simulink model "GolfSwing3D_KineticallyDrivenVariantSubsystems"  (R2024b)
settings: Solver=VariableStepAuto  StartTime=0.0  StopTime=StopTime  MaxStep=0.001  RelTol=1e-3
model workspace: external: MAT-File 3DModelInputs.mat (data not in the file)
undefined symbols (not defined in the file or in its folder): GripStrength, KillswitchFinalValue, KillswitchInitialValue, KillswitchStepTime, LeftLowerArmLength, PlaneTilt, RightLowerArmLength, UpperTorsoLength, X, Y, Z
libraries: nesl_utility x355, sm_lib x136, matrix_library x11, simulink x1
(part 1 of 13)
settings Model: Creator=dolso  LastModifiedBy=diete
settings SolverCC: MaxConsecutiveMinStep=20
settings DataIOCC: SaveOutput=off  SaveState=on
settings OptimizationCC: ReuseModelBlockBuffer=off
settings RTWCC: GPUComputeCapability=3.5
settings SimscapeCC: SimscapeLogType=all  SimscapeLogSimulationStatistics=on  SimscapeLogLimitData=off
settings ExplorerConfigSet: InternalSimMechanicsExplorerSettings="<ExplorerConfiguration><canonicalview>default</canonicalview><AnimationSetting><BasePlaybackSpeed>1.0</BasePlaybackSpeed><PlaybackSpeedFactor>1.0</PlaybackSpeedFactor></AnimationSetting><TilePanel><TileInfo><Tiles Columns=\"1\" Count=\"1\" Rows=\"1\"><Column Weight=\"1\"/><Row Weight=\"1\"/><Tile Height=\"1\" Width=\"1\" X=\"0\" Y=\"0\"/></Tiles></TileInfo><SceneInfo><SceneViewer><BGColor><R>0.800000011920928955</R><G>1</G><B>0.800000011920928955</B></BGColor><Camera><DoPerspective>off</DoPerspective><Position><X>0.223338250481492168</X><Y>-2.01724941781281597</Y><Z>0.561965888227227262</Z></Position><Center><X>0.223338250481492168</X><Y>-0.356681108474731556</Y><Z>0.561965888227227262</Z></Center><Up><X>0</X><Y>-0</Y><Z>1</Z></Up><ViewLimDist>1</ViewLimDist><YLim>1.48392906746005671</YLim><XLim>2.01139200613069313</XLim></Camera></SceneViewer></SceneInfo></TilePanel><MechEditorPanel><Cameras/><GfxPanelCameraMap/><VideoCreator><PlaybackSpeedRatio>1.0</PlaybackSpeedRatio><FrameRate>30</FrameRate><VideoFormat>Motion JPEG AVI</VideoFormat><FrameSize>auto</FrameSize></VideoCreator></MechEditorPanel></ExplorerConfiguration>"

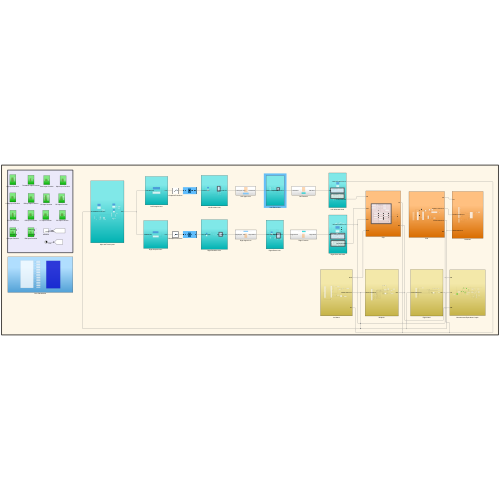
[thumbnail: Simulink's stored preview of the top-level diagram]
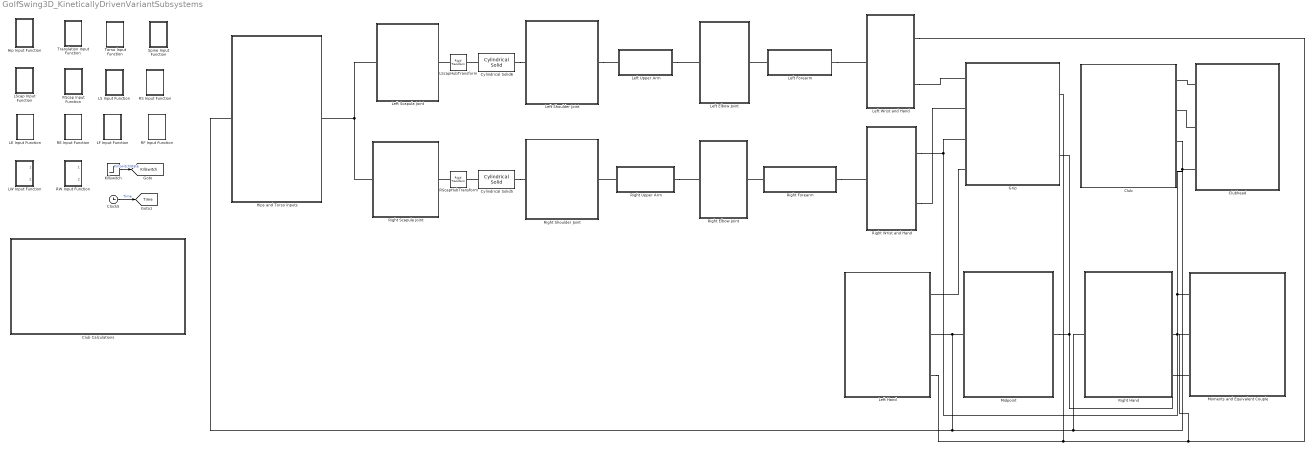
== system GolfSwing3D_KineticallyDrivenVariantSubsystems ==
  Clock5 : Clock
  Club : Subsystem
  Club Calculations : Subsystem
  Clubhead : Subsystem
  Cylindrical Solid5 : sm_lib/Body Elements/Cylindrical Solid  CylinderRadius=3  CylinderRadiusUnits=in  CylinderLength=10  CylinderLengthUnits=in  ExportEntireGeometry=off  InertiaType=CalculateFromGeometry  BasedOnType=Mass  Density=2000  DensityUnits=kg/m^3  Mass=10  MassUnits=kg  CenterOfMass=[0 0 0]  CenterOfMassUnits=m  MomentsOfInertia=[1 1 1]  MomentsOfInertiaUnits=kg*m^2  ProductsOfInertia=[0 0 0]  ProductsOfInertiaUnits=kg*m^2  GraphicType=FromGeometry  MarkerShape=Sphere  MarkerSize=10  GraphicVisPropType=SimpleVisualProperties  GraphicDiffuseColor=[0.2 0.2 1.0]  GraphicOpacity=1.0  GraphicSpecularColor=[0.5 0.5 0.5 1.0]  GraphicAmbientColor=[0.15 0.15 0.15 1.0]  GraphicEmissiveColor=[0.0 0.0 0.0 1.0]  GraphicShininess=75  DoExposeReferenceFrame=off  SerializedFrames=<Frames><Frame><Id>Frame1</Id><Value><Name>Hub</Name><Origin><Source>GeometricFeature</Source><FeatureName>top curve</FeatureName></Origin><PrimaryAxis><DefinedDirection>+X</DefinedDirection><Source>ReferenceFrame</Source><SourceDirection>-Z</SourceDirection><FeatureName></FeatureName></PrimaryAxis><SecondaryAxis><DefinedDirection>+Z</DefinedDirection><Source>ReferenceFrame</Source><SourceDirection>+Y</SourceDirection><FeatureName></FeatureName></SecondaryAxis></Value></Frame><Frame><Id>Frame2</Id><Value><Name>Right Shoulder</Name><Origin><Source>GeometricFeature</Source><FeatureName>bottom curve</FeatureName></Origin><PrimaryAxis><DefinedDirection>-X</DefinedDirection><Source>ReferenceFrame</Source><SourceDirection>+Z</SourceDirection><FeatureName></FeatureName></PrimaryAxis><SecondaryAxis><DefinedDirection>+Y</DefinedDirection><Source>ReferenceFrame</Source><SourceDirection>+X</SourceDirection><FeatureName></FeatureName></SecondaryAxis></Value></Frame></Frames>
  Cylindrical Solid6 : sm_lib/Body Elements/Cylindrical Solid  CylinderRadius=3  CylinderRadiusUnits=in  CylinderLength=10  CylinderLengthUnits=in  ExportEntireGeometry=off  InertiaType=CalculateFromGeometry  BasedOnType=Mass  Density=2000  DensityUnits=kg/m^3  Mass=10  MassUnits=kg  CenterOfMass=[0 0 0]  CenterOfMassUnits=m  MomentsOfInertia=[1 1 1]  MomentsOfInertiaUnits=kg*m^2  ProductsOfInertia=[0 0 0]  ProductsOfInertiaUnits=kg*m^2  GraphicType=FromGeometry  MarkerShape=Sphere  MarkerSize=10  GraphicVisPropType=SimpleVisualProperties  GraphicDiffuseColor=[0.2 0.2 1.0]  GraphicOpacity=1.0  GraphicSpecularColor=[0.5 0.5 0.5 1.0]  GraphicAmbientColor=[0.15 0.15 0.15 1.0]  GraphicEmissiveColor=[0.0 0.0 0.0 1.0]  GraphicShininess=75  DoExposeReferenceFrame=off  SerializedFrames=<Frames><Frame><Id>Frame1</Id><Value><Name>Hub</Name><Origin><Source>GeometricFeature</Source><FeatureName>top curve</FeatureName></Origin><PrimaryAxis><DefinedDirection>+X</DefinedDirection><Source>ReferenceFrame</Source><SourceDirection>-Z</SourceDirection><FeatureName></FeatureName></PrimaryAxis><SecondaryAxis><DefinedDirection>+Z</DefinedDirection><Source>ReferenceFrame</Source><SourceDirection>+Y</SourceDirection><FeatureName></FeatureName></SecondaryAxis></Value></Frame><Frame><Id>Frame2</Id><Value><Name>Left Shoulder</Name><Origin><Source>GeometricFeature</Source><FeatureName>bottom curve</FeatureName></Origin><PrimaryAxis><DefinedDirection>-X</DefinedDirection><Source>ReferenceFrame</Source><SourceDirection>+Z</SourceDirection><FeatureName></FeatureName></PrimaryAxis><SecondaryAxis><DefinedDirection>+Y</DefinedDirection><Source>ReferenceFrame</Source><SourceDirection>+X</SourceDirection><FeatureName></FeatureName></SecondaryAxis></Value></Frame></Frames>
  Grip : Subsystem
  Hip Input Function : Subsystem
  Hips and Torso Inputs : Subsystem
  Killswitch : Step  Time=KillswitchStepTime  Before=KillswitchInitialValue  After=KillswitchFinalValue  SampleTime=0
  LE Input Function : Subsystem
  LF Input Function : Subsystem
  LS Input Function : Subsystem
  LScap Input Function : Subsystem
  LScapHubTransform : sm_lib/Frames and Transforms/Rigid Transform  RotationMethod=RotationSequence  FollAlignAxisA=+X  BaseAlignAxisA=+Y  FollAlignAxisB=+Y  BaseAlignAxisB=+Z  RotationStandardAxis=+Z  RotationAngle=0  RotationAngleUnits=deg  RotationArbitraryAxis=[0 0 1]  RotationSequenceAxes=FollowerAxes  RotationSequence=ZXY  RotationSequenceAngles=[0 0 90]  RotationSequenceAnglesUnits=deg  RotationMatrix=[1 0 0;0 1 0;0 0 1]  Quaternion=[1 0 0 0]  TranslationMethod=None  TranslationCartesianOffset=[0 0 0]  TranslationCartesianOffsetUnits=m  TranslationStandardAxis=+Z  TranslationStandardOffset=0  TranslationStandardOffsetUnits=m  TranslationROffset=0  TranslationROffsetUnits=m  TranslationThetaOffset=0  TranslationThetaOffsetUnits=deg  TranslationZOffset=0  TranslationZOffsetUnits=m
  LW Input Function : Subsystem
  Left Elbow Joint : Subsystem
  Left Forearm : Subsystem
  Left Hand : Subsystem
  Left Scapula Joint : Subsystem
  Left Shoulder Joint : Subsystem
  Left Upper Arm : Subsystem
  Left Wrist and Hand : Subsystem
  Midpoint : Subsystem
  Moments and Equivalent Couple : Subsystem
  RE Input Function : Subsystem
  RF Input Function : Subsystem
  RS Input Function : Subsystem
  RScap Input Function : Subsystem
  RScapHubTransform : sm_lib/Frames and Transforms/Rigid Transform  RotationMethod=RotationSequence  FollAlignAxisA=+X  BaseAlignAxisA=+Y  FollAlignAxisB=+Y  BaseAlignAxisB=+Z  RotationStandardAxis=+Z  RotationAngle=0  RotationAngleUnits=deg  RotationArbitraryAxis=[0 0 1]  RotationSequenceAxes=FollowerAxes  RotationSequence=YXZ  RotationSequenceAngles=[-90 180 0]  RotationSequenceAnglesUnits=deg  RotationMatrix=[1 0 0;0 1 0;0 0 1]  Quaternion=[1 0 0 0]  TranslationMethod=None  TranslationCartesianOffset=[0 0 0]  TranslationCartesianOffsetUnits=m  TranslationStandardAxis=+Z  TranslationStandardOffset=0  TranslationStandardOffsetUnits=m  TranslationROffset=0  TranslationROffsetUnits=m  TranslationThetaOffset=0  TranslationThetaOffsetUnits=deg  TranslationZOffset=0  TranslationZOffsetUnits=m
  RW Input Function : Subsystem
  Right Elbow Joint : Subsystem
  Right Forearm : Subsystem
  Right Hand : Subsystem
  Right Scapula Joint : Subsystem
  Right Shoulder Joint : Subsystem
  Right Upper Arm : Subsystem
  Right Wrist and Hand : Subsystem
  Spine Input Function : Subsystem
  Torso Input Function : Subsystem
  Translation Input Function : Subsystem
  tag scope: Killswitch=global, Time=global
  wires:
  Clock5/1 -> [Time]  "Time"
  Killswitch/1 -> [Killswitch]  "KillswitchState"
  connections:
  Cylindrical Solid6/RConn1 -- Left Shoulder Joint/LConn1
  Left Scapula Joint/LConn1 -- Right Scapula Joint/LConn1 -- Hips and Torso Inputs/LConn1
  LScapHubTransform/LConn1 -- Left Scapula Joint/RConn1
  Cylindrical Solid5/LConn1 -- RScapHubTransform/RConn1
  RScapHubTransform/LConn1 -- Right Scapula Joint/RConn1
  Cylindrical Solid6/LConn1 -- LScapHubTransform/RConn1
  Cylindrical Solid5/RConn1 -- Right Shoulder Joint/LConn1
  Hips and Torso Inputs/RConn1 -- Club/RConn3 -- Clubhead/LConn3 -- Right Hand/LConn1 -- Left Hand/RConn2 -- Midpoint/LConn1
  Left Wrist and Hand/RConn1 -- Left Hand/RConn3 -- Grip/RConn1 -- Moments and Equivalent Couple/LConn2
  Right Wrist and Hand/RConn1 -- Club/RConn4 -- Moments and Equivalent Couple/LConn1 -- Right Hand/RConn1 -- Grip/LConn3
  Left Wrist and Hand/RConn2 -- Grip/LConn1
  Right Wrist and Hand/RConn2 -- Grip/LConn2
  Grip/LConn4 -- Left Hand/RConn1
  Clubhead/LConn1 -- Club/RConn1
  Clubhead/LConn2 -- Club/RConn2
  Midpoint/RConn1 -- Moments and Equivalent Couple/LConn3 -- Grip/RConn2
  Left Shoulder Joint/RConn1 -- Left Upper Arm/LConn1
  Left Upper Arm/RConn1 -- Left Elbow Joint/LConn1
  Left Forearm/LConn1 -- Left Elbow Joint/RConn1
  Left Forearm/RConn1 -- Left Wrist and Hand/LConn1
  Right Upper Arm/LConn1 -- Right Shoulder Joint/RConn1
  Right Upper Arm/RConn1 -- Right Elbow Joint/LConn1
  Right Forearm/LConn1 -- Right Elbow Joint/RConn1
  Right Forearm/RConn1 -- Right Wrist and Hand/LConn1

== system GolfSwing3D_KineticallyDrivenVariantSubsystems/Club ==
  Club COM : nesl_utility/PS-Simulink Converter  PhysicalDomain=network_engine_domain  SubClassName=ps_output  LeftPortType=input  RightPortType=output  PseudoPeriodic=off  Frequencies=[]  VectorFormat=1-D array  Unit=inherit  AffineConversion=off
  Club Mass : nesl_utility/PS-Simulink Converter  PhysicalDomain=network_engine_domain  SubClassName=ps_output  LeftPortType=input  RightPortType=output  PseudoPeriodic=off  Frequencies=[]  VectorFormat=1-D array  Unit=inherit  AffineConversion=off
  Clubface Vector : sm_lib/Body Elements/Cylindrical Solid  CylinderRadius=0.25  CylinderRadiusUnits=in  CylinderLength=CFVectorLength  CylinderLengthUnits=in  ExportEntireGeometry=off  InertiaType=CalculateFromGeometry  BasedOnType=Mass  Density=500  DensityUnits=kg/m^3  Mass=0  MassUnits=g  CenterOfMass=[0 0 0]  CenterOfMassUnits=m  MomentsOfInertia=[1 1 1]  MomentsOfInertiaUnits=kg*m^2  ProductsOfInertia=[0 0 0]  ProductsOfInertiaUnits=kg*m^2  GraphicType=FromGeometry  MarkerShape=Sphere  MarkerSize=10  GraphicVisPropType=SimpleVisualProperties  GraphicDiffuseColor=[0.4941 0.1843 0.5569]  GraphicOpacity=1.0  GraphicSpecularColor=[0.5 0.5 0.5 1.0]  GraphicAmbientColor=[0.15 0.15 0.15 1.0]  GraphicEmissiveColor=[0.0 0.0 0.0 1.0]  GraphicShininess=75  DoExposeReferenceFrame=off  SerializedFrames=<Frames><Frame><Id>Frame1</Id><Value><Name>Club Center</Name><Origin><Source>GeometricFeature</Source><FeatureName>top curve</FeatureName></Origin><PrimaryAxis><DefinedDirection>-Y</DefinedDirection><Source>ReferenceFrame</Source><SourceDirection>+Z</SourceDirection><FeatureName></FeatureName></PrimaryAxis><SecondaryAxis><DefinedDirection>+X</DefinedDirection><Source>ReferenceFrame</Source><SourceDirection>+Y</SourceDirection><FeatureName></FeatureName></SecondaryAxis></Value></Frame><Frame><Id>Frame2</Id><Value><Name>Center of Bottom</Name><Origin><Source>GeometricFeature</Source><FeatureName>bottom surface</FeatureName></Origin><PrimaryAxis><DefinedDirection>+Z</DefinedDirection><Source>ReferenceFrame</Source><SourceDirection>+Z</SourceDirection><FeatureName></FeatureName></PrimaryAxis><SecondaryAxis><DefinedDirection>+X</DefinedDirection><Source>ReferenceFrame</Source><SourceDirection>+X</SourceDirection><FeatureName></FeatureName></SecondaryAxis></Value></Frame></Frames>
  Clubhead : sm_lib/Body Elements/Spherical Solid  SphereRadius=ClubheadRadius  SphereRadiusUnits=in  ExportEntireGeometry=off  InertiaType=CalculateFromGeometry  BasedOnType=Mass  Density=500  DensityUnits=kg/m^3  Mass=0.25  MassUnits=kg  CenterOfMass=[0 0 0]  CenterOfMassUnits=m  MomentsOfInertia=[1 1 1]  MomentsOfInertiaUnits=kg*m^2  ProductsOfInertia=[0 0 0]  ProductsOfInertiaUnits=kg*m^2  GraphicType=FromGeometry  MarkerShape=Sphere  MarkerSize=10  GraphicVisPropType=SimpleVisualProperties  GraphicDiffuseColor=[0.0 0.0 0.0]  GraphicOpacity=1.0  GraphicSpecularColor=[0.5 0.5 0.5 1.0]  GraphicAmbientColor=[0.15 0.15 0.15 1.0]  GraphicEmissiveColor=[0.0 0.0 0.0 1.0]  GraphicShininess=75  DoExposeReferenceFrame=on  SerializedFrames=<Frames/>
  Flexible Beam Model : Subsystem
  ForceonClubhead : nesl_utility/PS-Simulink Converter  Commented=on  PhysicalDomain=network_engine_domain  SubClassName=ps_output  LeftPortType=input  RightPortType=output  PseudoPeriodic=off  Frequencies=[]  VectorFormat=1-D array  Unit=inherit  AffineConversion=off
  GripStrength : sm_lib/Frames and Transforms/Rigid Transform  RotationMethod=RotationSequence  FollAlignAxisA=+X  BaseAlignAxisA=+Y  FollAlignAxisB=+Y  BaseAlignAxisB=+Z  RotationStandardAxis=+Z  RotationAngle=0  RotationAngleUnits=deg  RotationArbitraryAxis=[0 0 1]  RotationSequenceAxes=FollowerAxes  RotationSequence=XYZ  RotationSequenceAngles=[-GripStrength 0 0]  RotationSequenceAnglesUnits=deg  RotationMatrix=[1 0 0;0 1 0;0 0 1]  Quaternion=[1 0 0 0]  TranslationMethod=None  TranslationCartesianOffset=[0 0 0]  TranslationCartesianOffsetUnits=m  TranslationStandardAxis=+Z  TranslationStandardOffset=0  TranslationStandardOffsetUnits=m  TranslationROffset=0  TranslationROffsetUnits=m  TranslationThetaOffset=0  TranslationThetaOffsetUnits=deg  TranslationZOffset=0  TranslationZOffsetUnits=m
  Inertia Sensor : sm_lib/Body Elements/Inertia Sensor  SensorExtent=BodyGroup  SpanWeldJoints=on  ExcludeGroundedBodies=off  MeasurementFrame=World  SenseMass=on  SenseCenterOfMass=on  SenseInertiaMatrix=on  SenseCenteredInertiaMatrix=off  SensePrincipalInertiaMatrix=off  SenseRotationMatrix=off  GraphicType=None  PrincipalInertiaFrameSize=20  GraphicVisPropType=SimpleVisualProperties  GraphicDiffuseColor=[0.5 0.5 0.5]  GraphicOpacity=1.0  GraphicSpecularColor=[0.5 0.5 0.5 1.0]  GraphicAmbientColor=[0.15 0.15 0.15 1.0]  GraphicEmissiveColor=[0.0 0.0 0.0 1.0]  GraphicShininess=75
  Rigid Shaft : Subsystem  Commented=on
  Weld Joint : sm_lib/Joints/Weld Joint  JointMode=Normal  CompositeWrenchDir=BaseOnFollower  CompositeWrenchFrame=BaseFrame  SenseConstraintForce=off  SenseConstraintTorque=off  SenseTotalForce=on  SenseTotalTorque=off
  Zero Mass Reference Shaft : Subsystem
  CH : PMIOPort  Side=Right
  Clubface Reference : PMIOPort  Port=2  Side=Right
  Global Reference : PMIOPort  Port=3  Side=Right
  RH : PMIOPort  Port=4  Side=Right
  tag scope: ClubCOM=global
  wires:
  Club COM/1 -> [ClubCOM]  "ClubCOM"
  ForceonClubhead/1 -> ?  "ForceonClubhead"
  connections:
  ForceonClubhead/LConn1 -- Weld Joint/RConn2
  Inertia Sensor/LConn1 -- CH/RConn1 -- Rigid Shaft/RConn2 -- Flexible Beam Model/RConn1 -- Weld Joint/LConn1
  Inertia Sensor/RConn1 -- Club Mass/LConn1
  Zero Mass Reference Shaft/RConn2 -- Global Reference/RConn1
  Club COM/LConn1 -- Inertia Sensor/RConn2
  GripStrength/LConn1 -- Weld Joint/RConn1
  Clubhead/RConn1 -- Clubface Vector/LConn1 -- GripStrength/RConn1
  Clubface Reference/RConn1 -- Clubface Vector/RConn1
  Zero Mass Reference Shaft/RConn1 -- Flexible Beam Model/LConn1 -- Rigid Shaft/RConn1 -- RH/RConn1

== system GolfSwing3D_KineticallyDrivenVariantSubsystems/Club Calculations ==
  Subsystem : Subsystem
  Work and Impulse Integrators : Subsystem
  tag scope: ForceAlongHandPath=global, ForceonClubMagnitude=global, HandForceYankLocal=global, LHForceAlongHandPath=global, LHonClubAngularPower=global, LHonClubLinearPower=global, LinearPoweronClub=global, RHForceAlongHandPath=global, RHonClubAngularPower=global, RHonClubLinearPower=global, SumofMomentsLHonClub=global, SumofMomentsRHonClub=global, TorqueonClubMagnitude=global, TotalHandForceGlobal=global, TotalHandForceLocal=global, TotalWristTorqueGlobal=global, TotalWristTorqueLocal=global
  wires:
  Subsystem/2(TotalHandTorqueLocal) -> [TotalWristTorqueLocal]  "TotalHandTorqueLocal"
  Subsystem/4(TotalHandTorqueGlobal) -> [TotalWristTorqueGlobal]  "TotalHandTorqueGlobal"
  Subsystem/1(TorqueonClubMagnitude) -> [TorqueonClubMagnitude]  "TorqueonClubMagnitude"
  Subsystem/3(TotalHandForceLocal) -> [TotalHandForceLocal]  "TotalHandForceLocal"
  Subsystem/5(TotalHandForceGlobal) -> [TotalHandForceGlobal]  "TotalHandForceGlobal"
  Subsystem/6(ForceonClubMagnitude) -> [ForceonClubMagnitude]  "ForceonClubMagnitude"
  Subsystem/7(HandForceYankLocal) -> [HandForceYankLocal]  "HandForceYankLocal"
  Subsystem/8(ForceAlongHandPath) -> [ForceAlongHandPath]  "ForceAlongHandPath"
  Subsystem/9(LinearPoweronClub) -> [LinearPoweronClub]  "LinearPoweronClub"
  Subsystem/10(LHonClubAngularPower) -> [LHonClubAngularPower]  "LHonClubAngularPower"
  Subsystem/11(RHonClubAngularPower) -> [RHonClubAngularPower]  "RHonClubAngularPower"
  Subsystem/12(SumofMomentsLHonClub) -> [SumofMomentsLHonClub]  "SumofMomentsLHonClub"
  Subsystem/13(SumofMomentsRHonClub) -> [SumofMomentsRHonClub]  "SumofMomentsRHonClub"
  Subsystem/14(LHonClubLinearPower) -> [LHonClubLinearPower]  "LHonClubLinearPower"
  Subsystem/15(RHonClubLinearPower) -> [RHonClubLinearPower]  "RHonClubLinearPower"
  Subsystem/16(LHForceAlongHandPath) -> [LHForceAlongHandPath]  "LHForceAlongHandPath"
  Subsystem/17(RHForceAlongHandPath) -> [RHForceAlongHandPath]  "RHForceAlongHandPath"

== system GolfSwing3D_KineticallyDrivenVariantSubsystems/Clubhead ==
  CH Unit Vector : MATLAB Function  TreatAsAtomicUnit=on  SystemSampleTime=0
  CHGlobalPosition : nesl_utility/PS-Simulink Converter  PhysicalDomain=network_engine_domain  SubClassName=ps_output  LeftPortType=input  RightPortType=output  PseudoPeriodic=off  Frequencies=[]  VectorFormat=1-D array  Unit=inherit  AffineConversion=off
  CHGlobalVelocity : nesl_utility/PS-Simulink Converter  PhysicalDomain=network_engine_domain  SubClassName=ps_output  LeftPortType=input  RightPortType=output  PseudoPeriodic=off  Frequencies=[]  VectorFormat=1-D array  Unit=inherit  AffineConversion=off
  Constant : Constant  Value=0
  MinMax Running Resettable : simulink/Math Operations/MinMax Running Resettable  Function=max  vinit=0.0
  TipPosition : nesl_utility/PS-Simulink Converter  PhysicalDomain=network_engine_domain  SubClassName=ps_output  LeftPortType=input  RightPortType=output  PseudoPeriodic=off  Frequencies=[]  VectorFormat=1-D array  Unit=inherit  AffineConversion=off
  Transform Sensor : sm_lib/Frames and Transforms/Transform Sensor  MeasurementFrame=World  RotationSequence=XYX  SenseAngle=off  SenseAxis=off  SenseQ=off  SenseR=off  SenseRotationSequence=off  SenseOmegaX=off  SenseOmegaY=off  SenseOmegaZ=off  SenseOmega=off  SenseQDot=off  SenseRDot=off  SenseRotationSequenceDot=off  SenseAlphaX=off  SenseAlphaY=off  SenseAlphaZ=off  SenseAlpha=off  SenseQDDot=off  SenseRDDot=off  SenseX=off  SenseY=off  SenseZ=off  SenseXYZ=on  SenseRad=off  SenseAzim=off  SenseDist=off  SenseInc=off  SenseXDot=off  SenseYDot=off  SenseZDot=off  SenseXYZDot=off  SenseRadDot=off  SenseAzimDot=off  SenseDistDot=off  SenseIncDot=off  SenseXDDot=off  SenseYDDot=off  SenseZDDot=off  SenseXYZDDot=off  SenseRadDDot=off  SenseAzimDDot=off  SenseDistDDot=off  SenseIncDDot=off
  Transform Sensor10 : sm_lib/Frames and Transforms/Transform Sensor  MeasurementFrame=World  RotationSequence=XYX  SenseAngle=off  SenseAxis=off  SenseQ=off  SenseR=off  SenseRotationSequence=off  SenseOmegaX=off  SenseOmegaY=off  SenseOmegaZ=off  SenseOmega=off  SenseQDot=off  SenseRDot=off  SenseRotationSequenceDot=off  SenseAlphaX=off  SenseAlphaY=off  SenseAlphaZ=off  SenseAlpha=off  SenseQDDot=off  SenseRDDot=off  SenseX=off  SenseY=off  SenseZ=off  SenseXYZ=on  SenseRad=off  SenseAzim=off  SenseDist=off  SenseInc=off  SenseXDot=off  SenseYDot=off  SenseZDot=off  SenseXYZDot=on  SenseRadDot=off  SenseAzimDot=off  SenseDistDot=off  SenseIncDot=off  SenseXDDot=off  SenseYDDot=off  SenseZDDot=off  SenseXYZDDot=off  SenseRadDDot=off  SenseAzimDDot=off  SenseDistDDot=off  SenseIncDDot=off
  CH : PMIOPort  Side=Left
  Clubface Reference : PMIOPort  Port=2  Side=Left
  Global Reference : PMIOPort  Port=3  Side=Left
  wires:
  TipPosition/1 -> CH Unit Vector/3(TipPosition)  "TipPosition"
  CHGlobalPosition/1 -> CH Unit Vector/1(CHGlobalPosition)  "CHGlobalPosition"
  CH Unit Vector/2(CHSpeedMPH) -> MinMax Running Resettable/1  "CHS (mph)"
  Constant/1 -> MinMax Running Resettable/2
  CHGlobalVelocity/1 -> CH Unit Vector/2(CHGlobalVelocity)  "CHy"
  connections:
  TipPosition/LConn1 -- Transform Sensor/RConn2
  Transform Sensor10/RConn1 -- CH/RConn1
  Transform Sensor/RConn1 -- Clubface Reference/RConn1
  CHGlobalVelocity/LConn1 -- Transform Sensor10/RConn3
  CHGlobalPosition/LConn1 -- Transform Sensor10/RConn2
  Transform Sensor/LConn1 -- Global Reference/RConn1 -- Transform Sensor10/LConn1
